simulink model "main_TDMA"  (R2017b)
settings: Solver=VariableStepAuto  StartTime=0.0  StopTime=10/fs  RelTol=1e-3
undefined symbols (not defined in the file): fs, gray
libraries: commdigbbndam3 x3, visionsources x2, commutil2 x2, commrflib2 x2, commsink2 x1
settings Model: Creator=changgang  LastModifiedBy=changgang

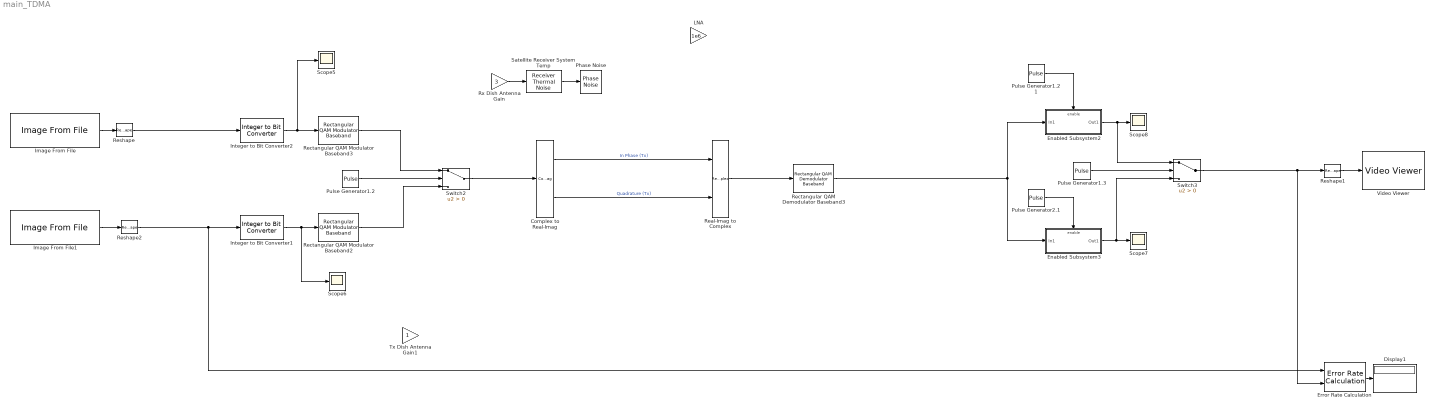
== system main_TDMA ==
  Complex to Real-Imag : ComplexToRealImag
  Display1 : Display
  Enabled Subsystem2 : Subsystem  TreatAsAtomicUnit=on
  Enabled Subsystem3 : Subsystem  TreatAsAtomicUnit=on
  Error Rate Calculation : commsink2/Error Rate Calculation  N=0  st_delay=0  cp_mode=Entire frame  subframe=[]  PMode=Port  WsName=ErrorVec  RsMode2=off  stop=off  numErr=100  maxBits=1e6
  Image From File : visionsources/Image From File  Tag=vipblks_nd  FileName=/Users/changgang/Documents/Changgang Zheng/Bachelor/Final Year 19-20/Winter Semester/Wireless and Optical Transmission Systems/Assignments/Matlab Code for Assignment/Figure/Asuka_2_value.png  imagePorts=One multidimensional signal  Ts=1/fs  ImageDataType=double  Signed=on  WordLength=16  sdImageDataType=uint(8)  FractionLengthMode=User-defined  FractionLength=15  OutPortLabels=G
      settings: SourceProductName=Computer Vision System Toolbox
  Image From File1 : visionsources/Image From File  Tag=vipblks_nd  FileName=/Users/changgang/Documents/Changgang Zheng/Bachelor/Final Year 19-20/Winter Semester/Wireless and Optical Transmission Systems/Assignments/Matlab Code for Assignment/Figure/Asuka_2_value.png  imagePorts=One multidimensional signal  Ts=1/fs  ImageDataType=double  Signed=on  WordLength=16  sdImageDataType=uint(8)  FractionLengthMode=User-defined  FractionLength=15  OutPortLabels=G
      settings: SourceProductName=Computer Vision System Toolbox
  Integer to Bit Converter1 : commutil2/Integer to Bit Converter  nbits=1  signedInputValues=Unsigned  bitOrder=LSB first  outDtype=boolean
  Integer to Bit Converter2 : commutil2/Integer to Bit Converter  nbits=1  signedInputValues=Unsigned  bitOrder=LSB first  outDtype=boolean
  LNA : Gain  Gain=1e6
  Phase Noise : commrflib2/Phase Noise  PhNs=-2  Fo=100  Fs=2e5  seed=2137
      settings: SourceProductName=Communications System Toolbox  SourceProductBaseCode=CM
  Pulse Generator1.2 : DiscretePulseGenerator  PulseType=Time based  Period=1/fs  PulseWidth=50
  Pulse Generator1.2 1 : DiscretePulseGenerator  PulseType=Time based  Period=1/fs  PulseWidth=50
  Pulse Generator1.3 : DiscretePulseGenerator  PulseType=Time based  Period=1/fs  PulseWidth=50
  Pulse Generator2.1 : DiscretePulseGenerator  PulseType=Time based  Period=1/fs  PulseWidth=50  PhaseDelay=0.05
  Real-Imag to Complex : RealImagToComplex
  Rectangular QAM Demodulator Baseband3 : commdigbbndam3/Rectangular QAM Demodulator Baseband  M=16  OutType=Bit  DecType=Hard decision  VarSource=Dialog  Variance=1  Dec=Gray  Mapping=[0:15]  PowType=Min. distance between symbols  MinDist=2  AvgPow=1  PeakPow=1  Ph=0  outDtype1=Inherit via internal rule  outDtype2=Inherit via internal rule  derotateFactorWordLen=16  derotateFactorDataTypeStr=Inherit: Same word length as input  derotateFactorLastDataTypeStr=Inherit: Same word length as input  denormFactorWordLen=16  denormFactorDataTypeStr=Inherit: Same word length as input  denormFactorLastDataTypeStr=Inherit: Same word length as input  prodOutWordLen=32  prodOutOverflowMode=Wrap  prodOutRoundingMode=Floor  prodOutOvFlMode=off  prodOutOvFlModeLastStrValue=off  sumWordLen=32
  Rectangular QAM Modulator Baseband2 : commdigbbndam3/Rectangular QAM Modulator Baseband  M=16  InType=Bit  Enc=Gray  Mapping=[0:15]  PowType=Min. distance between symbols  MinDist=2  AvgPow=1  PeakPow=1  Ph=0  outDtype=double  outWordLen=16  outUDDataType=sfix(16)  outFracLenMode=Best precision  outFracLen=15  outDataTypeStr=double  outLastDataTypeStr=double
  Rectangular QAM Modulator Baseband3 : commdigbbndam3/Rectangular QAM Modulator Baseband  M=16  InType=Bit  Enc=Gray  Mapping=[0:15]  PowType=Min. distance between symbols  MinDist=2  AvgPow=1  PeakPow=1  Ph=0  outDtype=double  outWordLen=16  outUDDataType=sfix(16)  outFracLenMode=Best precision  outFracLen=15  outDataTypeStr=double  outLastDataTypeStr=double
  Reshape : Reshape
  Reshape1 : Reshape  OutputDimensionality=Customize  OutputDimensions=[1050,700]
  Reshape2 : Reshape
  Rx Dish Antenna Gain : Gain  Gain=3  SaturateOnIntegerOverflow=on  OutDataTypeStr=Inherit: Same as input  ParamDataTypeStr=Inherit: Same as input
  Satellite Receiver System Temp : commrflib2/Receiver Thermal Noise  method=Noise temperature  ntemp=100  nfigure=20  nfactor=2  add290KAntennaNoise=off  seed=67987
      settings: SourceProductName=Communications System Toolbox  SourceProductBaseCode=CM
  Scope{5..8} (4 alike) : Scope
  Switch2 : Switch  Criteria=u2 > Threshold
  Switch3 : Switch  Criteria=u2 > Threshold
  Tx Dish Antenna Gain1 : Gain  SaturateOnIntegerOverflow=on  OutDataTypeStr=Inherit: Same as input  ParamDataTypeStr=Inherit: Same as input
  Video Viewer : VideoViewer  colormapValue=gray(256)  FigPos=[416 742 775 458]
  wires:
  Integer to Bit Converter2/1 -> Scope5/1, Rectangular QAM Modulator Baseband3/1
  Rectangular QAM Modulator Baseband2/1 -> Switch2/3
  Reshape1/1 -> Video Viewer/1
  Reshape/1 -> Integer to Bit Converter2/1
  Pulse Generator1.2 1/1 -> Enabled Subsystem2/Enable
  Rectangular QAM Modulator Baseband3/1 -> Switch2/1
  Pulse Generator1.2/1 -> Switch2/2
  Image From File1/1 -> Reshape2/1
  Integer to Bit Converter1/1 -> Scope6/1, Rectangular QAM Modulator Baseband2/1
  Image From File/1 -> Reshape/1
  Enabled Subsystem2/1(Out1) -> Switch3/1, Scope8/1
  Rectangular QAM Demodulator Baseband3/1 -> Enabled Subsystem3/1(In1), Enabled Subsystem2/1(In1)
  Enabled Subsystem3/1(Out1) -> Switch3/3, Scope7/1
  Switch3/1 -> Error Rate Calculation/2, Reshape1/1
  Pulse Generator2.1/1 -> Enabled Subsystem3/Enable
  Pulse Generator1.3/1 -> Switch3/2
  Complex to Real-Imag/1 -> Real-Imag to Complex/1  "In Phase (Tx)"
  Complex to Real-Imag/2 -> Real-Imag to Complex/2  "Quadrature (Tx)"
  Rx Dish Antenna Gain/1 -> Satellite Receiver System Temp/1
  Satellite Receiver System Temp/1 -> Phase Noise/1
  Error Rate Calculation/1 -> Display1/1
  Reshape2/1 -> Error Rate Calculation/1, Integer to Bit Converter1/1
  Real-Imag to Complex/1 -> Rectangular QAM Demodulator Baseband3/1
  Switch2/1 -> Complex to Real-Imag/1

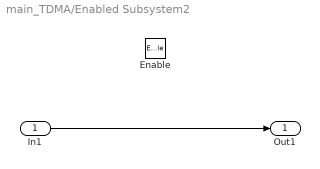
== system main_TDMA/Enabled Subsystem2 ==
  In1 : Inport
  Enable : EnablePort
  Out1 : Outport
  wires:
  In1/1 -> Out1/1

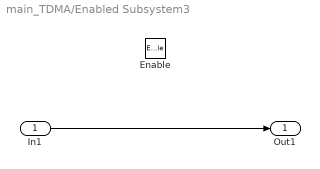
== system main_TDMA/Enabled Subsystem3 ==
  In1 : Inport
  Enable : EnablePort
  Out1 : Outport
  wires:
  In1/1 -> Out1/1
